simulink model "ModelNieLiniowy"  (R2014a)
settings: Solver=ode45  StartTime=0.0  StopTime=10  MinStep=0.1  RelTol=1e-3
values from neighbouring files (symbols this model uses):
  K0 = lqr(A0,B0,Q0,R0)    [WyznaczanieParametrow.m]
  K30 = lqr(A30,B30,Q30,R30)    [WyznaczanieParametrow.m]
libraries: fuzblock x1
settings Model: Creator=Szwank  LastModifiedBy=Szwank

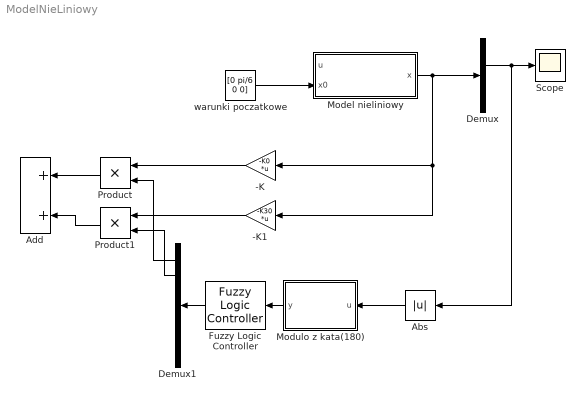
== system ModelNieLiniowy ==
  -K : Gain  Gain=-K0  Multiplication=Matrix(K*u)
  -K1 : Gain  Gain=-K30  Multiplication=Matrix(K*u)
  Abs : Abs
  Add : Sum
  Demux : Demux
  Demux1 : Demux  Outputs=7
  Fuzzy Logic Controller : fuzblock/Fuzzy Logic  Controller  fis='modelRozmyty.fis'
  "Model nieliniowy " : Subsystem
  Modulo z kata(180) : MATLAB Function  TreatAsAtomicUnit=on
  Product : Product
  Product1 : Product
  Scope : Scope
      settings: YMin=4.665  YMax=4.76
  warunki poczatkowe : Constant  Value=[0 pi/6 0 0]
  wires:
  warunki poczatkowe/1 -> "Model nieliniowy "/2(x0)
  "Model nieliniowy "/1(x) -> -K1/1, -K/1, Demux/1
  Demux/2 -> Abs/1, Scope/1
  Fuzzy Logic Controller/1 -> Demux1/1
  Abs/1 -> Modulo z kata(180)/1(u)
  Modulo z kata(180)/1(y) -> Fuzzy Logic Controller/1
  -K/1 -> Product/1
  Demux1/1 -> Product/2
  Demux1/2 -> Product1/2
  -K1/1 -> Product1/1
  Product/1 -> Add/1
  Product1/1 -> Add/2

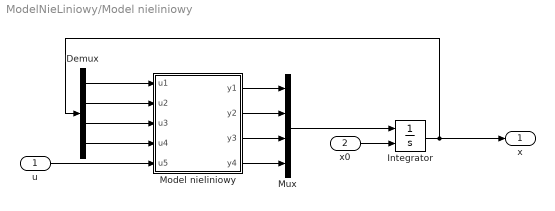
== system ModelNieLiniowy/Model nieliniowy  ==
  "u " : Inport
  x0 : Inport  Port=2
  Demux : Demux
  Integrator : Integrator  InitialConditionSource=external
  Model nieliniowy : MATLAB Function  TreatAsAtomicUnit=on
  Mux : Mux
  x : Outport
  wires:
  Demux/1 -> Model nieliniowy/1(u1)
  Demux/2 -> Model nieliniowy/2(u2)
  Demux/3 -> Model nieliniowy/3(u3)
  Demux/4 -> Model nieliniowy/4(u4)
  Mux/1 -> Integrator/1
  Model nieliniowy/1(y1) -> Mux/1
  Model nieliniowy/2(y2) -> Mux/2
  Model nieliniowy/3(y3) -> Mux/3
  Model nieliniowy/4(y4) -> Mux/4
  Integrator/1 -> x/1, Demux/1
  x0/1 -> Integrator/2
  "u "/1 -> Model nieliniowy/5(u5)

== matlab function ModelNieLiniowy/Model nieliniowy /Model nieliniowy ==
  data: u1 input; y1 output; u2 input; u3 input; u4 input; u5 input; y2 output; y3 output; y4 output
function [y1,y2,y3,y4] = fcn(u1,u2,u3,u4,u5)
%Dane obiektu
%% Motor
Rm = 3.3; % ohms, Motor armature resistance 
Kt = 0.0280; % N.m, Motor torque constant
Km = 0.0280; % V/(rad/s), Motor back-emf constant (same as Ktin SI units)
Jm = 9.64e-6; % kg.m2, Moment of inertia of motor rotor. 
Jeq = 1.23e-4; % kg.m2, Equivalent moment of inertia about motor shaft pivot axis.
%% Pendulum Arm:
Marm = 0.0280; % kg, Mass of the arm.
r = 0.0826; % m, Length of arm pivot to pendulum pivot.
Beq = 0.01; % N.m/(rad/s), Arm viscous damping. 
%% Pendulum Link:
Mp = 0.0270; % kg, Mass of the pendulum link and weight combined.
Lp = 0.191; % m, Total length of pendulum.
lp = 0.153; % m, Length of pendulum center of mass from pivot.
Jp = 1.20e-4; % kg.m2, Pendulum moment of inertia about its pivot axis.
Bp = 0; % N.m/(rad/s), Pendulum viscous damping.
%% Pulse-Width Modulated Amplifier:
Vmax = 24; % V, PWM amplifier maximum output voltage
PWM = 5; % A, amplifier maximum output current
Kw = 2.3; % V/V, PWM amplifier gain
%% Stałe
m = Mp;
g = 9.80665;
a = Jeq + m * r^2;
b = m * lp * r;
e = m*lp^2 + Jp;
f = m*g*lp;
c = Km*Kw/Rm;
d = (Km*Kt+Beq*Rm)/Rm;
%%

y1 = u3;
y2 = u4;
y3 = 1/(1-(b^2/(a*e))*cos(u2)^2)*(1/a)*(b*f/e*sin(u2)*cos(u2)-b*u4^2*sin(u2)+u5*c-d*u3);
y4 = 1/(1-(b^2/(a*e))*cos(u2)^2)*(1/e)*(b/a*cos(u2)*(-b*u4^2*sin(u2)+c*u5-d*u3)+f*sin(u2));

== matlab function ModelNieLiniowy/Modulo z kata(180) ==
  data: u input; y output
function y = fcn(u)
%#codegen

y = u;
